simulink model "evaluate_noise_model"  (R2023b)
settings: Solver=VariableStepAuto  StartTime=0.0  StopTime=24  FixedStep=1  RelTol=1e-3
undefined symbols (not defined in the file or in its folder): ks, Ts
settings Model: Creator=hdt  LastModifiedBy=hdt

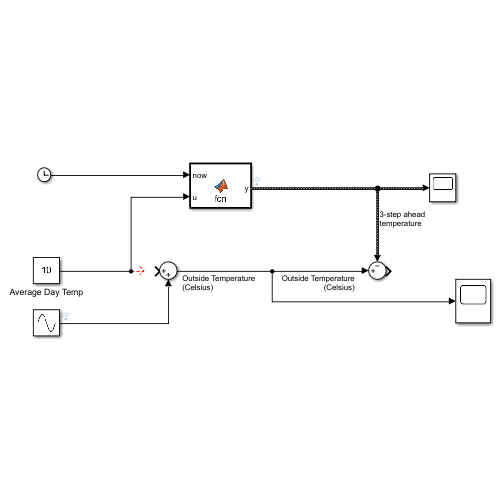
[thumbnail: Simulink's stored preview of the top-level diagram]
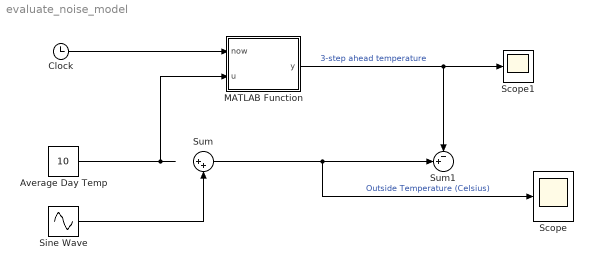
== system evaluate_noise_model ==
  Average Day Temp : Constant  Value=10
  Clock : Clock
  MATLAB Function : MATLAB Function  TreatAsAtomicUnit=on
  Scope : Scope
  Scope1 : Scope
  Sine Wave : Sin  Amplitude=4  Bias=10  Frequency=pi/12  SampleTime=0
  Sum : Sum  Inputs=|++
  Sum1 : Sum  Inputs=-+|
  wires:
  Average Day Temp/1 -> MATLAB Function/2(u)
  Sine Wave/1 -> Sum/2
  Sum/1 -> Scope/1, Sum1/2  "Outside Temperature (Celsius)"
  Clock/1 -> MATLAB Function/1(now)
  MATLAB Function/1(y) -> Scope1/1, Sum1/1  "3-step ahead temperature"

== matlab function evaluate_noise_model/MATLAB Function ==
  settings: updateMethod=DISCRETE  sampleTime=1
  data: now input; u input; y output size=horizon; ks parameter; Ts parameter
function y = fcn(now, u, ks, Ts)
    y = 4*sin(pi/12 .* (now + ks*Ts) + 0) + u;
end
